simulink model "sampleModel127"  (R2021b)
settings: Solver=VariableStepAuto  StartTime=0.0  StopTime=10.0  RelTol=1e-3
undefined symbols (not defined in the file or in its folder): DiscIntNeverNeededParam, Newton, Raphson
libraries: simulink x5, slpidlib x1
settings Model: Creator=user  LastModifiedBy=user

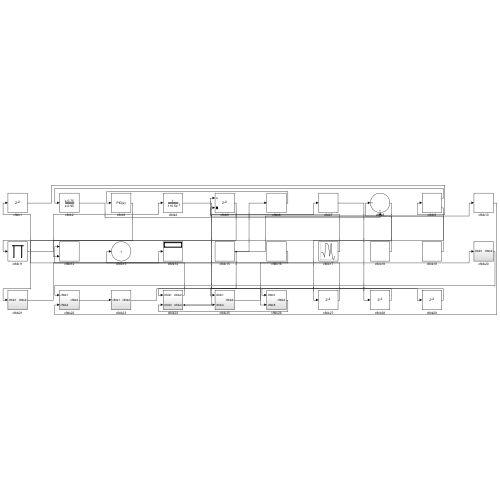
[thumbnail: Simulink's stored preview of the top-level diagram]
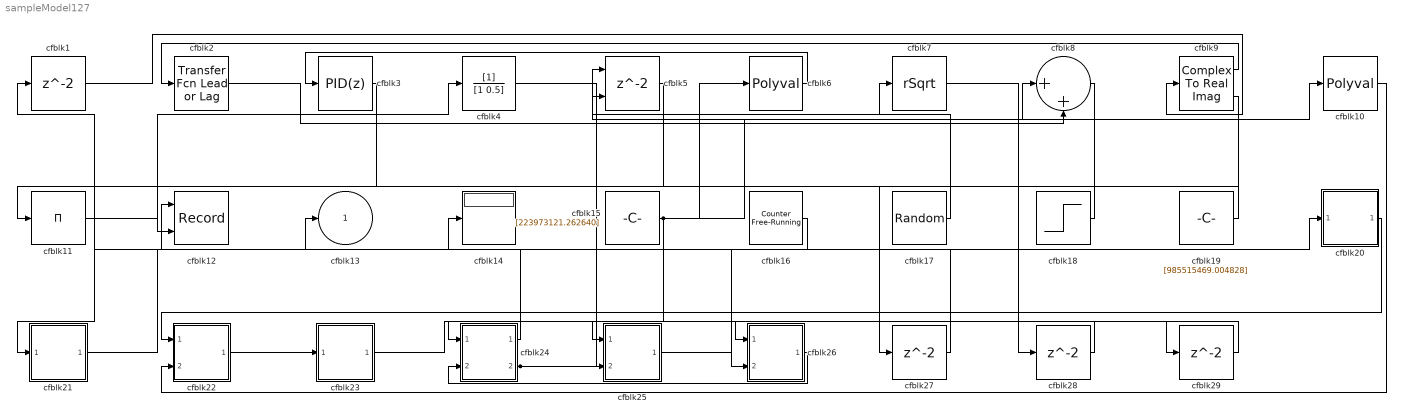
== system sampleModel127 ==
  cfblk{1,27..29} (4 alike) : Delay  SampleTime=1
  cfblk10 : Polyval  Coefs=[ +2.081618890e-019, -1.441693666e-014, +4.719686976e-010, -8.536869453e-006, +1.621573104e-001, -8.087801117e+001 ]
  cfblk11 : Product  Inputs=*
  cfblk12 : Record  FileSettingsInternal="{\"entries\":[{\"content\":{\"excelSettings\":{\"content\":{},\"type\":\"Streamout.ExcelSettings\"}},\"type\":\"Streamout.FileSettingStorage\",\"uuid\":\"7024c3bf-7f11-4887-85ee-93702250b512\"}],\"packageUris\":[\"http://schema.mathworks.com/mf0/streamout_blocks/R2020a\"],\"version\":\"1.0\"}"  Layout=[1 1]  SignalsInternal="{\"entries\":[{\"content\":{\"signals\":[{\"content\":{\"blockPath\":[\"sampleModel127/cfblk12\"],\"channel\":[],\"dimensions\":[1],\"domain\":\"sampleModel127/cfblk12\",\"lineColor\":\"#a2142f\",\"plots\":[1],\"port\":1,\"sid\":[\"\"],\"signalID\":4470,\"signalName\":\"cfblk16\"},\"type\":\"RecordBlkView.Signal\",\"uuid\":\"529234e9-00a4-43e7-a067-70c9af3e3ba2\"},{\"content\":{\"blockPath\":[\"sampleModel127/cfblk12\"],\"channel\":[],\"dimensions\":[1],\"domain\":\"sampleModel127/cfblk12\",\"lineColor\":\"#139fff\",\"plots\":[1],\"port\":2,\"sid\":[\"\"],\"signalID\":4474,\"signalName\":\"cfblk5\"},\"type\":\"RecordBlkView.Signal\",\"uuid\":\"33b3caa4-e488-406d-9d3d-7be28a48f812\"}]},\"type\":\"RecordBlkView.InputSignals\",\"uuid\":\"d7d82b3f-b0a8-4a43-9b30-81c9bed282a0\"}],\"packageUris\":[\"http://schema.mathworks.com/mf0/streamout_blocks/R2020a\"],\"version\":\"1.0\"}"  VisualizationBindings="{\"xyplotplugin\":{\"info\":[{\"series\":[{\"bindingParametersList\":[{\"parameter\":\"X-Axis\",\"signalID\":4470,\"signalName\":\"cfblk16\"},{\"parameter\":\"Y-Axis\",\"signalID\":4474,\"signalName\":\"cfblk5\"}],\"seriesID\":40513}],\"subplotID\":1}]}}"  CompatibilityTag=XY
  cfblk14 : Display
  cfblk15 : Constant  Value=[223973121.262640]  SampleTime=1
  cfblk16 : simulink/Sources/Counter Free-Running  NumBits=[25.000000]  tsamp=-1
  cfblk17 : RandomNumber  Mean=[16997.686069]  Variance=[35356.770147]  Seed=[398324829.000000]  SampleTime=0.1
  cfblk18 : Step  Time=[1.000000]  Before=[350593096.515837]  After=[849369577.227583]  SampleTime=0
  cfblk19 : Constant  Value=[985515469.004828]  SampleTime=1
  cfblk2 : simulink/Discrete/Transfer Fcn Lead or Lag  PoleZ=0.95  ZeroZ=0.75  ICPrevOutput=0.0  ICPrevInput=0.0  DoSatur=off
      settings: SourceProductBaseCode=SL
  cfblk20 : Subsystem
  cfblk21 : Subsystem
  cfblk22 : Subsystem
  cfblk23 : Subsystem
  cfblk24 : Subsystem
  cfblk25 : Subsystem
  cfblk26 : Subsystem
  cfblk3 : slpidlib/PID Controller  Controller=PID  Form=Parallel  TimeDomain=Discrete-time  UseExternalTs=off  SampleTime=1  IntegratorMethod=Forward Euler  FilterMethod=Forward Euler  ControllerParametersSource=internal  P=1  I=1  D=0  UseFilter=on  N=100  TunerSelectOption=Transfer Function Based (PID Tuner App)  InitialConditionSource=internal  InitialConditionForIntegrator=0  InitialConditionForFilter=0  DifferentiatorICPrevScaledInput=0  ExternalReset=none  TrackingMode=off  Kt=1  LimitOutput=off  SatLimitsSource=internal  UpperSaturationLimit=inf  LowerSaturationLimit=-inf  LinearizeAsGain=off  AntiWindupMode=none  Kb=1  POutMin=[]  POutMax=[]  IOutMin=[]  IOutMax=[]  DOutMin=[]  DOutMax=[]  NOutMin=[]  NOutMax=[]  SumOutMin=[]  SumOutMax=[]  SaturationOutMin=[]  SaturationOutMax=[]  PParamMin=[]  PParamMax=[]  IParamMin=[]  IParamMax=[]  DParamMin=[]  DParamMax=[]  NParamMin=[]  NParamMax=[]  KbParamMin=[]  KbParamMax=[]  KtParamMin=[]  KtParamMax=[]  KbOutMin=[]  KbOutMax=[]  KtOutMin=[]  KtOutMax=[]  IntegratorOutMin=[]  IntegratorOutMax=[]  FilterOutMin=[]  FilterOutMax=[]  SumI1OutMin=[]  SumI1OutMax=[]  SumI2OutMin=[]  SumI2OutMax=[]  SumI3OutMin=[]  SumI3OutMax=[]  SumI4OutMin=[]  SumI4OutMax=[]  SumDOutMin=[]  SumDOutMax=[]  DifferentiatorOutMin=[]  DifferentiatorOutMax=[]  FilterDiffOutCoefMin=[]  FilterDiffOutCoefMax=[]  ReciprocalOutMin=[]  ReciprocalOutMax=[]  SumDenOutMin=[]  SumDenOutMax=[]  SumNumOutMin=[]  SumNumOutMax=[]  DivideOutMin=[]  DivideOutMax=[]  UdiffTsProdOutMin=[]  UdiffTsProdOutMax=[]  NTsProdOutMin=[]  NTsProdOutMax=[]  UintegralTsProdOutMin=[]  UintegralTsProdOutMax=[]  UngainTsProdOutMin=[]  UngainTsProdOutMax=[]  IntegratorContinuousStateAttributes=''  IntegratorStateMustResolveToSignalObject=off  IntegratorRTWStateStorageClass=Auto  FilterContinuousStateAttributes=''  FilterStateMustResolveToSignalObject=off  FilterRTWStateStorageClass=Auto  ParallelPVariant=InternalParameters  IdealPVariant=Disabled  IVariant=InternalParameters  DVariant=InternalParameters  IntegratorVariant=Discrete  SatVariant=Disabled  AWVariant=Passthrough  PCopyVariant=Disabled  TRVariant=Disabled  FdbkBlocksVariant=Forward  IdealPFdbkVariant=Disabled  SatFdbkVariant=Disabled  DerivativeFilterVariant=ForwardEulerFilter  NVariant=InternalParameters  NCopyVariant=Disabled  FilterICVariant=InternalICsFilter  IntegratorICVariant=InternalICs  ExternalResetVariant=Disabled  TRSumVariant=Passthrough  SumFdbkVariant=Disabled  SumVariant=Sum_PID  TsampFilterVariant=InternalTs  TsampNgainVariant=Passthrough  TsampIntegralVariant=Passthrough  ExternalSaturationOutDataTypeStr=Inherit: Same as second input
  cfblk4 : DiscreteFilter  SampleTime=1
  cfblk5 : Delay  ShowEnablePort=on  SampleTime=1
      settings: InputPortMap=u0,e6
  cfblk6 : Polyval  Coefs=[ +2.081618890e-019, -1.441693666e-014, +4.719686976e-010, -8.536869453e-006, +1.621573104e-001, -8.087801117e+001 ]
  cfblk7 : Sqrt  Operator=rSqrt  AlgorithmType=Newton-Raphson  SaturateOnIntegerOverflow=on
  cfblk8 : Sum  Inputs=|++
  cfblk9 : ComplexToRealImag
  cfblk13 : Outport
  wires:
  cfblk15/1 -> cfblk10/1, cfblk25/1(cfblk1), cfblk6/1
  cfblk16/1 -> cfblk12/1
  cfblk6/1 -> cfblk3/1
  cfblk3/1 -> cfblk11/1
  cfblk17/1 -> cfblk5/1
  cfblk20/1(cfblk2) -> cfblk22/1(cfblk1)
  cfblk9/1 -> cfblk2/1
  cfblk5/1 -> cfblk12/2
  cfblk25/1(cfblk2) -> cfblk20/1(cfblk1)
  cfblk24/1(cfblk2) -> cfblk13/1
  cfblk4/1 -> cfblk26/2(cfblk5)
  cfblk1/1 -> cfblk9/1
  cfblk18/1 -> cfblk5/2
  cfblk26/1(cfblk2) -> cfblk24/2(cfblk3)
  cfblk24/2(cfblk4) -> cfblk7/1, cfblk25/2(cfblk4)
  cfblk22/1(cfblk2) -> cfblk23/1(cfblk1)
  cfblk8/1 -> cfblk21/1(cfblk1)
  cfblk21/1(cfblk2) -> cfblk14/1
  cfblk19/1 -> cfblk8/1
  cfblk2/1 -> cfblk8/2
  cfblk10/1 -> cfblk22/2(cfblk4)
  cfblk11/1 -> cfblk4/1
  cfblk9/2 -> cfblk27/1
  cfblk27/1 -> cfblk1/1
  cfblk7/1 -> cfblk28/1
  cfblk28/1 -> cfblk24/1(cfblk1)
  cfblk23/1(cfblk2) -> cfblk29/1
  cfblk29/1 -> cfblk26/1(cfblk1)

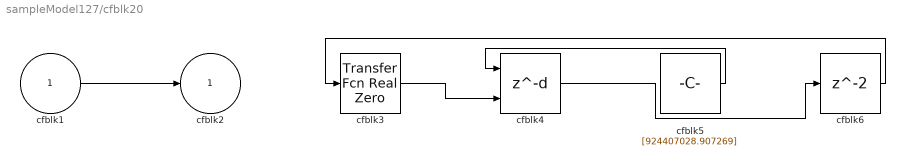
== system sampleModel127/cfblk20 ==
  cfblk1 : Inport
  cfblk3 : simulink/Discrete/Transfer Fcn Real Zero  ZeroZ=0.75  ICPrevInput=0.0  DoSatur=off
      settings: SourceProductBaseCode=SL
  cfblk4 : Delay  DelayLengthSource=Input port  SampleTime=1
      settings: InputPortMap=u0,p1
  cfblk5 : Constant  Value=[924407028.907269]  SampleTime=1
  cfblk6 : Delay  SampleTime=1
  cfblk2 : Outport
  wires:
  cfblk5/1 -> cfblk4/1
  cfblk1/1 -> cfblk2/1
  cfblk3/1 -> cfblk4/2
  cfblk4/1 -> cfblk6/1
  cfblk6/1 -> cfblk3/1

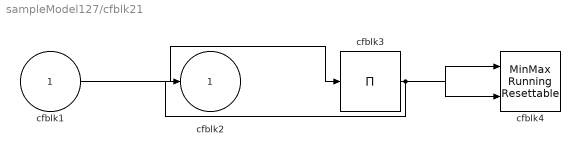
== system sampleModel127/cfblk21 ==
  cfblk1 : Inport
  cfblk3 : Product  Inputs=*
  cfblk4 : simulink/Math Operations/MinMax Running Resettable  Function=min  vinit=0.0
  cfblk2 : Outport
  wires:
  cfblk1/1 -> cfblk3/1
  cfblk3/1 -> cfblk2/1, cfblk4/1, cfblk4/2

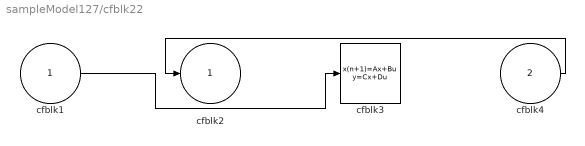
== system sampleModel127/cfblk22 ==
  cfblk1 : Inport
  cfblk4 : Inport  Port=2
  cfblk3 : DiscreteStateSpace
  cfblk2 : Outport
  wires:
  cfblk4/1 -> cfblk2/1
  cfblk1/1 -> cfblk3/1

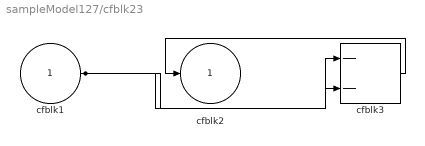
== system sampleModel127/cfblk23 ==
  cfblk1 : Inport
  cfblk3 : Sum  Inputs=--
  cfblk2 : Outport
  wires:
  cfblk3/1 -> cfblk2/1
  cfblk1/1 -> cfblk3/1, cfblk3/2

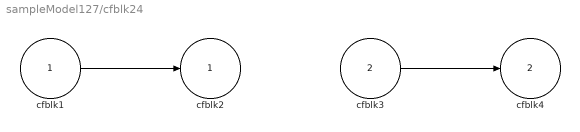
== system sampleModel127/cfblk24 ==
  cfblk1 : Inport
  cfblk3 : Inport  Port=2
  cfblk2 : Outport
  cfblk4 : Outport  Port=2
  wires:
  cfblk1/1 -> cfblk2/1
  cfblk3/1 -> cfblk4/1

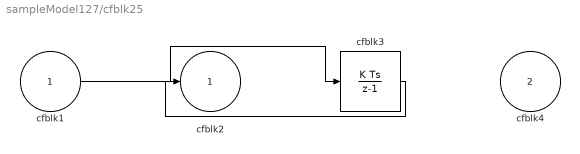
== system sampleModel127/cfblk25 ==
  cfblk1 : Inport
  cfblk4 : Inport  Port=2
  cfblk3 : DiscreteIntegrator  ICPrevOutput=DiscIntNeverNeededParam  ICPrevScaledInput=DiscIntNeverNeededParam
  cfblk2 : Outport
  wires:
  cfblk1/1 -> cfblk3/1
  cfblk3/1 -> cfblk2/1

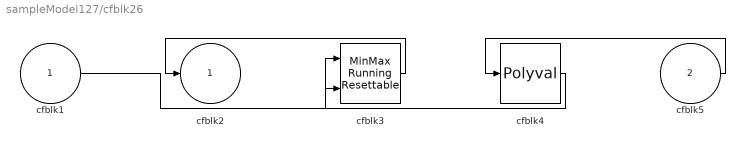
== system sampleModel127/cfblk26 ==
  cfblk1 : Inport
  cfblk5 : Inport  Port=2
  cfblk3 : simulink/Math Operations/MinMax Running Resettable  Function=min  vinit=0.0
  cfblk4 : Polyval  Coefs=[ +2.081618890e-019, -1.441693666e-014, +4.719686976e-010, -8.536869453e-006, +1.621573104e-001, -8.087801117e+001 ]
  cfblk2 : Outport
  wires:
  cfblk3/1 -> cfblk2/1
  cfblk5/1 -> cfblk4/1
  cfblk4/1 -> cfblk3/1
  cfblk1/1 -> cfblk3/2
